simulink model "quadrotor_stage4_waypoints"  (R2026a)
settings: Solver=ode4  StartTime=0  StopTime=30  FixedStep=0.005  MaxStep=0.005  RelTol=1e-6
undefined symbols (not defined in the file): DiscIntNeverNeededParam
settings Model: Creator=ASUS  LastModifiedBy=ASUS

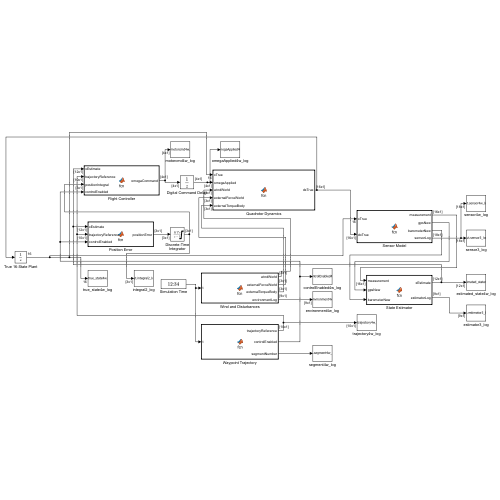
[thumbnail: Simulink's stored preview of the top-level diagram]
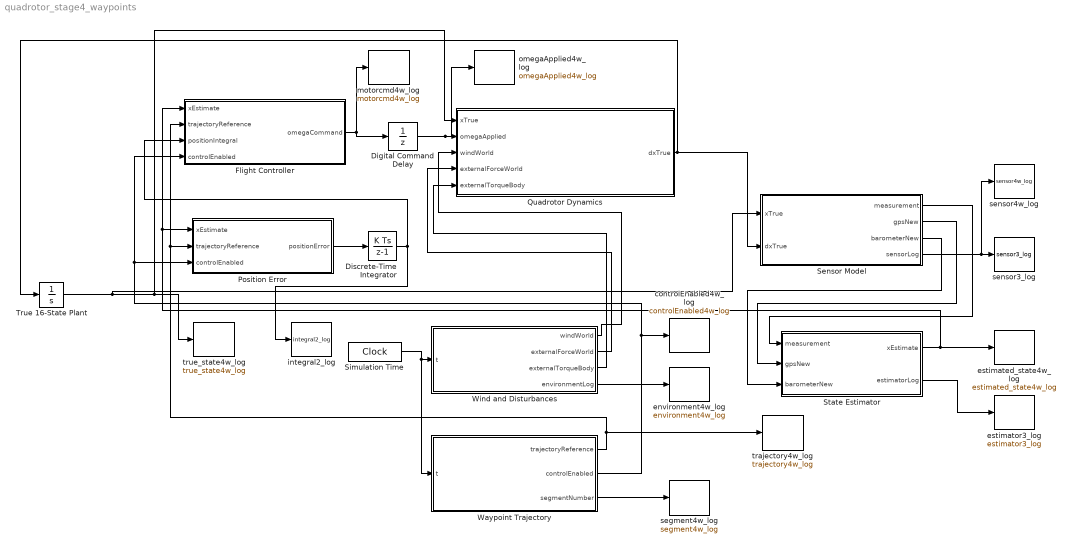
== system quadrotor_stage4_waypoints ==
  Digital Command Delay : UnitDelay  InitialCondition=sqrt(1.20*9.81/(4*1.8e-5))*ones(4,1)  SampleTime=0.005
  Discrete-Time Integrator : DiscreteIntegrator  InitialCondition=zeros(3,1)  SampleTime=0.005  LimitOutput=on  UpperSaturationLimit=[4;4;1.5]  LowerSaturationLimit=[-4;-4;-1.5]  ICPrevOutput=DiscIntNeverNeededParam  ICPrevScaledInput=DiscIntNeverNeededParam
  Flight Controller : MATLAB Function  TreatAsAtomicUnit=on
  Position Error : MATLAB Function  TreatAsAtomicUnit=on
  Quadrotor Dynamics : MATLAB Function  TreatAsAtomicUnit=on
  Sensor Model : MATLAB Function  TreatAsAtomicUnit=on
  Simulation Time : DigitalClock
  State Estimator : MATLAB Function  TreatAsAtomicUnit=on
  True 16-State Plant : Integrator  InitialCondition=[zeros(12,1); sqrt(1.20*9.81/(4*1.8e-5))*ones(4,1)]
  Waypoint Trajectory : MATLAB Function  TreatAsAtomicUnit=on
  Wind and Disturbances : MATLAB Function  TreatAsAtomicUnit=on
  controlEnabled4w_log : ToWorkspace  VariableName=controlEnabled4w_log  SaveFormat=Timeseries  SampleTime=-1
      settings: Save2DSignal=2-D array (concatenate along first dimension)
  environment4w_log : ToWorkspace  VariableName=environment4w_log  SaveFormat=Timeseries  SampleTime=-1
      settings: Save2DSignal=2-D array (concatenate along first dimension)
  estimated_state4w_log : ToWorkspace  VariableName=estimated_state4w_log  SaveFormat=Timeseries  SampleTime=-1
      settings: Save2DSignal=2-D array (concatenate along first dimension)
  estimator3_log : ToWorkspace  VariableName=estimator3_log  SaveFormat=Timeseries  SampleTime=-1
      settings: Save2DSignal=2-D array (concatenate along first dimension)
  integral2_log : ToWorkspace  VariableName=integral2_log  SaveFormat=Timeseries  SampleTime=-1
      settings: Save2DSignal=2-D array (concatenate along first dimension)
  motorcmd4w_log : ToWorkspace  VariableName=motorcmd4w_log  SaveFormat=Timeseries  SampleTime=-1
      settings: Save2DSignal=2-D array (concatenate along first dimension)
  omegaApplied4w_log : ToWorkspace  VariableName=omegaApplied4w_log  SaveFormat=Timeseries  SampleTime=-1
      settings: Save2DSignal=2-D array (concatenate along first dimension)
  segment4w_log : ToWorkspace  VariableName=segment4w_log  SaveFormat=Timeseries  SampleTime=-1
      settings: Save2DSignal=2-D array (concatenate along first dimension)
  sensor3_log : ToWorkspace  VariableName=sensor3_log  SaveFormat=Timeseries  SampleTime=-1
      settings: Save2DSignal=2-D array (concatenate along first dimension)
  sensor4w_log : ToWorkspace  VariableName=sensor4w_log  SaveFormat=Timeseries  SampleTime=-1
      settings: Save2DSignal=2-D array (concatenate along first dimension)
  trajectory4w_log : ToWorkspace  VariableName=trajectory4w_log  SaveFormat=Timeseries  SampleTime=-1
      settings: Save2DSignal=2-D array (concatenate along first dimension)
  true_state4w_log : ToWorkspace  VariableName=true_state4w_log  SaveFormat=Timeseries  SampleTime=-1
      settings: Save2DSignal=2-D array (concatenate along first dimension)
  wires:
  Flight Controller/1(omegaCommand) -> motorcmd4w_log/1, Digital Command Delay/1
  True 16-State Plant/1 -> Sensor Model/1(xTrue), true_state4w_log/1, Quadrotor Dynamics/1(xTrue)
  Position Error/1(positionError) -> Discrete-Time Integrator/1
  Discrete-Time Integrator/1 -> integral2_log/1, Flight Controller/3(positionIntegral)
  Simulation Time/1 -> Waypoint Trajectory/1(t), Wind and Disturbances/1(t)
  Wind and Disturbances/1(windWorld) -> Quadrotor Dynamics/3(windWorld)
  Wind and Disturbances/2(externalForceWorld) -> Quadrotor Dynamics/4(externalForceWorld)
  Wind and Disturbances/3(externalTorqueBody) -> Quadrotor Dynamics/5(externalTorqueBody)
  Wind and Disturbances/4(environmentLog) -> environment4w_log/1
  Quadrotor Dynamics/1(dxTrue) -> True 16-State Plant/1, Sensor Model/2(dxTrue)
  Sensor Model/1(measurement) -> State Estimator/1(measurement)
  Sensor Model/2(gpsNew) -> State Estimator/2(gpsNew)
  Sensor Model/3(barometerNew) -> State Estimator/3(barometerNew)
  State Estimator/1(xEstimate) -> estimated_state4w_log/1, Position Error/1(xEstimate), Flight Controller/1(xEstimate)
  Waypoint Trajectory/1(trajectoryReference) -> Position Error/2(trajectoryReference), Flight Controller/2(trajectoryReference), trajectory4w_log/1
  Waypoint Trajectory/2(controlEnabled) -> Position Error/3(controlEnabled), Flight Controller/4(controlEnabled), controlEnabled4w_log/1
  Digital Command Delay/1 -> omegaApplied4w_log/1, Quadrotor Dynamics/2(omegaApplied)
  State Estimator/2(estimatorLog) -> estimator3_log/1
  Sensor Model/4(sensorLog) -> sensor4w_log/1, sensor3_log/1
  Waypoint Trajectory/3(segmentNumber) -> segment4w_log/1

== matlab function quadrotor_stage4_waypoints/Quadrotor Dynamics ==
  data: xTrue input; dxTrue output; omegaApplied input; windWorld input; externalForceWorld input; externalTorqueBody input
function dxTrue = fcn(xTrue, omegaApplied, windWorld, ...
    externalForceWorld, externalTorqueBody)
%#codegen

dxTrue = zeros(16,1);

dxTrue = quadDynamicsStage3( ...
    xTrue, omegaApplied, windWorld, ...
    externalForceWorld, externalTorqueBody);
end

== matlab function quadrotor_stage4_waypoints/Flight Controller ==
  settings: updateMethod=DISCRETE  sampleTime=0.005
  data: xEstimate input; omegaCommand output; trajectoryReference input; positionIntegral input; controlEnabled input
function omegaCommand = fcn(xEstimate, trajectoryReference, ...
    positionIntegral, controlEnabled)
%#codegen

omegaCommand = zeros(4,1);

omegaCommand = flightControllerStage4Waypoints( ...
    xEstimate, trajectoryReference, ...
    positionIntegral, controlEnabled);
end

== matlab function quadrotor_stage4_waypoints/Position Error ==
  settings: updateMethod=DISCRETE  sampleTime=0.005
  data: xEstimate input; positionError output; trajectoryReference input; controlEnabled input
function positionError = fcn(xEstimate, trajectoryReference, controlEnabled)
%#codegen

positionError = zeros(3,1);
if controlEnabled(1)
    positionError(1) = trajectoryReference(1)-xEstimate(1);
    positionError(2) = trajectoryReference(2)-xEstimate(2);
    positionError(3) = trajectoryReference(3)-xEstimate(3);
end
end

== matlab function quadrotor_stage4_waypoints/Wind and Disturbances ==
  data: t input; windWorld output; externalForceWorld output; externalTorqueBody output; environmentLog output
function [windWorld, externalForceWorld, ...
    externalTorqueBody, environmentLog] = fcn(t)
%#codegen

windWorld = zeros(3,1);
externalForceWorld = zeros(3,1);
externalTorqueBody = zeros(3,1);
environmentLog = zeros(9,1);
end

== matlab function quadrotor_stage4_waypoints/Waypoint Trajectory ==
  data: t input; trajectoryReference output; controlEnabled output; segmentNumber output
function [trajectoryReference, controlEnabled, segmentNumber] = fcn(t)
%#codegen

trajectoryReference = zeros(10,1);
controlEnabled = false;
segmentNumber = 0.0;

[generatedReference, generatedEnable, generatedSegment] = ...
    waypointTrajectoryStage4(t(1));

trajectoryReference(1:10) = generatedReference(1:10);
controlEnabled = generatedEnable(1);
segmentNumber = generatedSegment(1);
end

== matlab function quadrotor_stage4_waypoints/Sensor Model ==
  settings: updateMethod=DISCRETE  sampleTime=0.005
  data: xTrue input; measurement output; dxTrue input; gpsNew output; barometerNew output; sensorLog output
function [measurement, gpsNew, barometerNew, sensorLog] = ...
    fcn(xTrue, dxTrue)
%#codegen
[measurement, gpsNew, barometerNew, sensorLog] = ...
    sensorModelStage3(xTrue, dxTrue);
end

== matlab function quadrotor_stage4_waypoints/State Estimator ==
  settings: updateMethod=DISCRETE  sampleTime=0.005
  data: measurement input; xEstimate output; gpsNew input; barometerNew input; estimatorLog output
function [xEstimate, estimatorLog] = ...
    fcn(measurement, gpsNew, barometerNew)
%#codegen

[xEstimate, estimatorLog] = stateEstimatorStage3( ...
    measurement, gpsNew, barometerNew);
end
